simulink model "nms_3Dmodel_forward"  (R2017b)
settings: Solver=VariableStepAuto  StartTime=0.0  StopTime=t_end  FixedStep=1e-4  MinStep=1e-9  RelTol=1e-2  AbsTol=1e-3  EnableMultiTasking=on
InitFcn:
  | runScripts;
values from neighbouring files (symbols this model uses):
  ankle_height = 0.08    [nms_MechInit.m]
  ankleIMP = param(91+length(paramIC_opt):93+length(paramIC_opt))    [runScripts.m]
  c = 0.05    [IID_nms_MechInit.m]    (also in nms_MechInit.m)
  c_jointstop = 0.3 / (pi/180)    (= 17.1887338539)    [IID_nms_MechInit.m]    (also in nms_MechInit.m)
  CPG_On = 0    [setCPGPar.m]    (also in setCPGPar_inv.m = 1)
  CtrlPar_FP = [alpha0 alpha_cd alpha_cv]    [setCtrlPar.m]
  CtrlPar_FP_R = [R_hipR0 R_hipR_cd R_hipR_cv]    [setCtrlPar.m]
  CtrlPar_LL = l_clr    [setCtrlPar.m]
  CtrlPar_Side = [beta_cd  beta_cv]    [setCtrlPar.m]
  CtrlPar_St = [StPreStim St_M1 St_M2 St_M3 St_M4 St_M5 St_M11]    [setCtrlPar.m]
  CtrlPar_St_R = [R_StPreStim R_St_M1 R_St_M3 R_St_M4]    [setCtrlPar.m]
  CtrlPar_Sw = [SwPreStim SwPhasePari SwPhaseParii SwCtrlPar_H SwCtrlPar_A      SwCtrlPar_Ki SwCtrlPar_Kii SwCtrlPar_Kiii SwCtrlPar_StP]    [setCtrlPar.m]
  CtrlPar_Sw_R = [R_SwPreStim R_Sw_M6]    [setCtrlPar.m]
  CtrlPar_theta0 = parBlCtrl(1)      *1*pi/180    [setCtrlPar.m]
  CtrlPar_Tr = [Tr_St_sup Tr_Sw]    [setCtrlPar.m]
  CtrlPar_Tr_R = [R_Tr_St_sup R_Tr_Sw]    [setCtrlPar.m]
  D12_F = 0.16    [IID_nms_MechInit.m]    (also in nms_MechInit.m)
  D12_S = L_S    (= 0.5)    [IID_nms_MechInit.m]    (also in nms_MechInit.m = 0.46)
  D12_T = L_T    (= 0.5)    [IID_nms_MechInit.m]    (also in nms_MechInit.m = 0.46)
  D12z_T = 0.1* scalorFactor    (= 0.1)    [nms_MechInit.m]
  D13_F = 0.20    (= 0.2)    [IID_nms_MechInit.m]    (also in nms_MechInit.m)
  D1G_F = 0.14    [IID_nms_MechInit.m]    (also in nms_MechInit.m)
  D1G_HAT = 0.35    [IID_nms_MechInit.m]    (also in nms_MechInit.m)
  D1G_S = 0.3    [IID_nms_MechInit.m]    (also in nms_MechInit.m = 0.28)
  D1G_T = 0.3    [IID_nms_MechInit.m]    (also in nms_MechInit.m = 0.28)
  D1Gy_F = ankle_height*D1G_F/D12_F    (= 0.07)    [nms_MechInit.m]
  d_fBall = 0.1    [nms_MechInit.m]
  d_fHeel = 0.05    [nms_MechInit.m]
  DeltaThRef = 5e-3    (= 0.005)    [IID_nms_MechInit.m]    (also in nms_MechInit.m)
  Dist_LM23_PH = 0    [setDistPar.m]
  Dist_LM34_PH = 0    [setDistPar.m]
  Dist_On = 1    [IID_setDistPar.m]    (also in setDistPar.m)
  Dist_PDur = 0.15    [IID_setDistPar.m]    (also in setDistPar.m)
  Dist_RM23_PH = 0    [setDistPar.m]
  Dist_RM34_PH = 0    [setDistPar.m]
  Dist_StartTime = 15    [IID_setDistPar.m]    (also in setDistPar.m)
  Dist_xyzHAT_front_PH = 0    [setDistPar.m]
  Dist_xyzHAT_sag_PH = 0    [IID_setDistPar.m]    (also in setDistPar.m)
  Dist_xyzLAnkle_PH = 0    [setDistPar.m]
  Dist_xyzRAnkle_PH = 0    [setDistPar.m]
  eref = 0.04    [IID_nms_MechInit.m]    (also in nms_MechInit.m)
  FmaxBFSH = 350    [nms_MechInit.m]
  FmaxGAS = 1500    [IID_nms_MechInit.m]    (also in nms_MechInit.m)
  FmaxGLU = 1500    [IID_nms_MechInit.m]    (also in nms_MechInit.m)
  FmaxHAB = 3000    [nms_MechInit.m]
  FmaxHAD = 4500    [nms_MechInit.m]
  FmaxHAM = 3000    [IID_nms_MechInit.m]    (also in nms_MechInit.m)
  FmaxHFL = 2000    [IID_nms_MechInit.m]    (also in nms_MechInit.m)
  FmaxRF = 1200    [nms_MechInit.m]
  FmaxSOL = 4000    [IID_nms_MechInit.m]    (also in nms_MechInit.m)
  FmaxTA = 800    [IID_nms_MechInit.m]    (also in nms_MechInit.m)
  FmaxVAS = 6000    [IID_nms_MechInit.m]    (also in nms_MechInit.m)
  In_F = 0.005    [IID_nms_MechInit.m]    (also in nms_MechInit.m)
  In_HAT = 3    [IID_nms_MechInit.m]    (also in nms_MechInit.m = 2.5)
  In_S = 0.05    [IID_nms_MechInit.m]    (also in nms_MechInit.m)
  In_T = 0.15    [IID_nms_MechInit.m]    (also in nms_MechInit.m)
  init_a_tgt = 70*pi/180    (= 1.2217304764)    [setInitPar.m]
  init_a_tgtR = 90*pi/180    (= 1.57079632679)    [setInitPar.m]
  Inx_F = 0.0007    [nms_MechInit.m]
  Inx_HAT = 1.0    (= 1)    [nms_MechInit.m]
  Inx_S = 0.003    [nms_MechInit.m]
  Inx_T = 0.03    [nms_MechInit.m]
  Iny_F = 0.005    [nms_MechInit.m]
  Iny_HAT = 4.0    (= 4)    [nms_MechInit.m]
  Iny_S = 0.05    [nms_MechInit.m]
  Iny_T = 0.15    [nms_MechInit.m]
  K = 5    [IID_nms_MechInit.m]    (also in nms_MechInit.m)
  k_gn = k_gn/2    (= 39240)    [nms_MechInit.m]
  k_gt = k_gt/2    (= 3924)    [nms_MechInit.m]
  k_pressure = m_HAT * 9.81 / DeltaThRef    (= 104967)    [IID_nms_MechInit.m]    (also in nms_MechInit.m)
  leg_l = [D12_T D12_S]    [nms_MechInit.m]
  LongDelay = 0.020    (= 0.02)    [IID_setCtrlPar.m]    (also in nms_MechInit.m = 0.01)
  LongLoopDelay = 0.030    (= 0.03)    [nms_MechInit.m]
  loptBFSH = 0.12    [nms_MechInit.m]
  loptGAS = 0.05    [IID_nms_MechInit.m]    (also in nms_MechInit.m)
  loptGLU = 0.11    [IID_nms_MechInit.m]    (also in nms_MechInit.m)
  loptHAB = 0.09    [nms_MechInit.m]
  loptHAD = 0.10    (= 0.1)    [nms_MechInit.m]
  loptHAM = 0.10    (= 0.1)    [IID_nms_MechInit.m]    (also in nms_MechInit.m)
  loptHFL = 0.11    [IID_nms_MechInit.m]    (also in nms_MechInit.m)
  loptRF = 0.08    [nms_MechInit.m]
  loptSOL = 0.04    [IID_nms_MechInit.m]    (also in nms_MechInit.m)
  loptTA = 0.06    [IID_nms_MechInit.m]    (also in nms_MechInit.m)
  loptVAS = 0.08    [IID_nms_MechInit.m]    (also in nms_MechInit.m)
  lslackBFSH = 0.10    (= 0.1)    [nms_MechInit.m]
  lslackGAS = 0.40    (= 0.4)    [IID_nms_MechInit.m]    (also in nms_MechInit.m)
  lslackGLU = 0.13    [IID_nms_MechInit.m]    (also in nms_MechInit.m)
  lslackHAB = 0.07    [nms_MechInit.m]
  lslackHAD = 0.18    [nms_MechInit.m]
  lslackHAM = 0.31    [IID_nms_MechInit.m]    (also in nms_MechInit.m)
  lslackHFL = 0.10    (= 0.1)    [IID_nms_MechInit.m]    (also in nms_MechInit.m)
  lslackRF = 0.35    [nms_MechInit.m]
  lslackSOL = 0.26    [IID_nms_MechInit.m]    (also in nms_MechInit.m)
  lslackTA = 0.24    [IID_nms_MechInit.m]    (also in nms_MechInit.m)
  lslackVAS = 0.23    [IID_nms_MechInit.m]    (also in nms_MechInit.m)
  m_F = 1.25    [IID_nms_MechInit.m]    (also in nms_MechInit.m)
  m_HAT = 53.5    [IID_nms_MechInit.m]    (also in nms_MechInit.m)
  m_S = 3.5    [IID_nms_MechInit.m]    (also in nms_MechInit.m)
  m_T = 8.5    [IID_nms_MechInit.m]    (also in nms_MechInit.m)
  m_Total = m_F*2+m_S*2+m_T*2+m_HAT    (= 80)    [IID_nms_MechInit.m]    (also in nms_MechInit.m)
  massBFSH = 2    [nms_MechInit.m]
  massGAS = 0.45    [IID_nms_MechInit.m]    (also in nms_MechInit.m)
  massGLU = 1.4    [IID_nms_MechInit.m]    (also in nms_MechInit.m)
  massHAB = 1.145    [nms_MechInit.m]
  massHAD = 1.91    [nms_MechInit.m]
  massHAM = 1.82    [IID_nms_MechInit.m]    (also in nms_MechInit.m)
  massHFL = 1.87    [IID_nms_MechInit.m]    (also in nms_MechInit.m)
  massRF = 1    [nms_MechInit.m]
  massSOL = 1.36    [IID_nms_MechInit.m]    (also in nms_MechInit.m)
  massTA = 0.29    [IID_nms_MechInit.m]    (also in nms_MechInit.m)
  massVAS = 2.91    [IID_nms_MechInit.m]    (also in nms_MechInit.m)
  MidDelay = 0.010    (= 0.01)    [IID_setCtrlPar.m]    (also in nms_MechInit.m = 0.005)
  mu_slide = 0.8    [IID_nms_MechInit.m]    (also in nms_MechInit.m)
  mu_stick = 0.9    [IID_nms_MechInit.m]    (also in nms_MechInit.m)
  N = 1.5    [IID_nms_MechInit.m]    (also in cmaes_parfor.m = size(x,1); nms_MechInit.m)
  phi12_LowLimit = 70*pi/180    (= 1.2217304764)    [IID_nms_MechInit.m]    (also in nms_MechInit.m)
  phi12_UpLimit = 130*pi/180    (= 2.26892802759)    [IID_nms_MechInit.m]    (also in nms_MechInit.m)
  phi23_UpLimit = 175*pi/180    (= 3.05432619099)    [IID_nms_MechInit.m]    (also in nms_MechInit.m)
  phi34_UpLimit = 230*pi/180    (= 4.01425727959)    [IID_nms_MechInit.m]    (also in nms_MechInit.m)
  phi34R_LowLimit = -15*pi/180    (= -0.261799387799)    [nms_MechInit.m]
  ... (+115 more)
undefined symbols (not defined in the file or in its folder): Control_type, Fs_prosthesis, magnitude, sgn
libraries: mblibv1 x104, simulink x54, simulink_extras x38, nmc x30, NMCCPG_Library x17, powerlib_meascontrol x5
(part 3 of 17)

== system nms_3Dmodel_forward/CPG ==
  note: CPG State Observer
      | Learning Center
      | Learns the signals of all sensors
      | If signals are prelearned, only loads the signals
      |
      | CPG Output
      | Estimates rate of change (roc at all instances of various time model
      | Becomes active after signals are saved or loaded
      |
      | Saver
      | Saves signals to workspace after learning is done
      |
      | Etc
      | Creates signals necessary in CPG model
  CPG Output : Subsystem
  Etc : Subsystem
  Learning center : Subsystem
  Saver : Subsystem  Commented=on

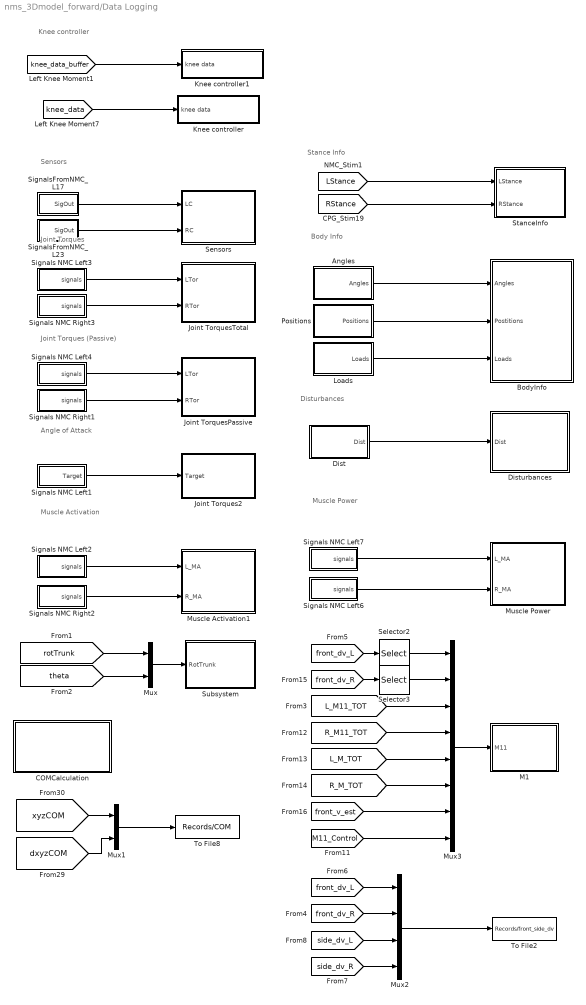
== system nms_3Dmodel_forward/Data Logging ==
  note: Sensors
  note: Stance Info
  note: Muscle Activation
  note: Joint Torques
  note: Disturbances
  note: Angle of Attack
  note: Body Info
  note: Joint Torques (Passive)
  note: Muscle Power
  note: Knee controller
  Angles : Subsystem
  BodyInfo : Subsystem
  "COMCalculation " : Subsystem
  Dist : Subsystem
  Disturbances : Subsystem
  Joint Torques2 : Subsystem
  Joint TorquesPassive : Subsystem
  Joint TorquesTotal : Subsystem
  Knee controller : Subsystem
  Knee controller1 : Subsystem
  Loads : Subsystem
  M1 : Subsystem
  Muscle Activation1 : Subsystem
  Muscle Power : Subsystem
  Mux : Mux  Inputs=2
  Mux1 : Mux  Inputs=2
  Mux2 : Mux
  Mux3 : Mux  Inputs=8
  Positions : Subsystem
  Selector2 : Selector  InputPortWidth=2  IndexOptions=Index vector (dialog)  Indices=[2]  OutputSizes=1
  Selector3 : Selector  InputPortWidth=2  IndexOptions=Index vector (dialog)  Indices=[2]  OutputSizes=1
  Sensors : Subsystem
  Signals NMC Left1 : Subsystem
  Signals NMC Left2 : Subsystem
  Signals NMC Left3 : Subsystem
  Signals NMC Left4 : Subsystem
  Signals NMC Left6 : Subsystem
  Signals NMC Left7 : Subsystem
  Signals NMC Right1 : Subsystem
  Signals NMC Right2 : Subsystem
  Signals NMC Right3 : Subsystem
  SignalsFromNMC_L17 : Subsystem  mask{LorR='L', Add=''}
      mask prompts: LorR "Right or Left"; Add "Addition"
      mask init:
      | blk = gcb;
      | set_param([gcb '/From'],'GotoTag',[LorR,'FmGLU',Add]);
      | set_param([gcb '/From1'],'GotoTag',[LorR,'FmHAM',Add]);
      | set_param([gcb '/From2'],'GotoTag',[LorR,'FmVAS',Add]);
      | set_param([gcb '/From3'],'GotoTag',[LorR,'LceBFSH',Add]);
      | set_param([gcb '/From4'],'GotoTag',[LorR,'FmGAS',Add]);
      | 
      | set_param([gcb '/From5'],'GotoTag',[LorR,'FmSOL',Add]);
      | set_param([gcb '/From6'],'GotoTag',[LorR,'LceTA',Add]);
      | set_param([gcb '/From7'],'GotoTag',[LorR,'LceRF',Add]);
      | set_param([gcb '/From8'],'GotoTag',[LorR,'VceRF',Add]);
      | set_param([gcb '/From9'],'GotoTag',[LorR,'LceHAM',Add]);
      | 
      | set_param([gcb '/From10'],'GotoTag',[LorR,'VceHAM',Add]);
      | set_param([gcb '/From11'],'GotoTag',[LorR,'VceVAS',Add]);
      | set_param([gcb '/From12'],'GotoTag',[LorR,'VceBFSH',Add]);
      | set_param([gcb '/From13'],'GotoTag',[LorR,'LceHFL',Add]);
      | set_param([gcb '/From14'],'GotoTag',[LorR,'LceGLU',Add]);
      | 
      | set_param([gcb '/From15'],'GotoTag',[LorR,'LceVAS',Add]);
      | set_param([gcb '/From16'],'GotoTag',[LorR,'FmHAB',Add]);
      | set_param([gcb '/From17'],'GotoTag',[LorR,'LceHAD',Add]);
      | set_param([gcb '/From18'],'GotoTag',[LorR,'LceHAB',Add]);
  SignalsFromNMC_L23 : Subsystem  mask{LorR='R', Add=''}
      mask prompts: LorR "Right or Left"; Add "Addition"
      mask init: same as nms_3Dmodel_forward/Data Logging/SignalsFromNMC_L17
  StanceInfo : Subsystem
  Subsystem : Subsystem
  To File2 : ToFile  Filename=Records/front_side_dv
  To File8 : ToFile  Filename=Records/COM
  wires:
  SignalsFromNMC_L17/1(SigOut) -> Sensors/1(LC)
  SignalsFromNMC_L23/1(SigOut) -> Sensors/2(RC)
  Signals NMC Right2/1(signals) -> Muscle Activation1/2(R_MA)
  Signals NMC Left2/1(signals) -> Muscle Activation1/1(L_MA)
  Signals NMC Left3/1(signals) -> Joint TorquesTotal/1(LTor)
  Signals NMC Right3/1(signals) -> Joint TorquesTotal/2(RTor)
  Angles/1(Angles) -> BodyInfo/1(Angles)
  Positions/1(Positions) -> BodyInfo/2(Postitions)
  [LStance] -> StanceInfo/1(LStance)
  [RStance] -> StanceInfo/2(RStance)
  Loads/1(Loads) -> BodyInfo/3(Loads)
  Signals NMC Left1/1(Target) -> Joint Torques2/1(Target)
  Dist/1(Dist) -> Disturbances/1(Dist)
  [rotTrunk] -> Mux/1
  [theta] -> Mux/2
  Signals NMC Left4/1(signals) -> Joint TorquesPassive/1(LTor)
  Signals NMC Right1/1(signals) -> Joint TorquesPassive/2(RTor)
  Signals NMC Left6/1(signals) -> Muscle Power/2(R_MA)
  Signals NMC Left7/1(signals) -> Muscle Power/1(L_MA)
  Mux/1 -> Subsystem/1(RotTrunk)
  [dxyzCOM] -> Mux1/2
  [xyzCOM] -> Mux1/1
  Mux1/1 -> To File8/1
  Selector2/1 -> Mux3/1
  [front_dv_L] -> Selector2/1
  [L_M_TOT] -> Mux3/5
  [R_M_TOT] -> Mux3/6
  [L_M11_TOT] -> Mux3/3
  [R_M11_TOT] -> Mux3/4
  [front_dv_R] -> Selector3/1
  Selector3/1 -> Mux3/2
  Mux3/1 -> M1/1(M11)
  [M11_Control] -> Mux3/8
  [front_v_est] -> Mux3/7
  [side_dv_R] -> Mux2/4
  [front_dv_R] -> Mux2/2
  [side_dv_L] -> Mux2/3
  [front_dv_L] -> Mux2/1
  Mux2/1 -> To File2/1
  [knee_data] -> Knee controller/1(knee data)
  [knee_data_buffer] -> Knee controller1/1(knee data)

== system nms_3Dmodel_forward/Disturbances ==
  Clock : Clock
  Compare To Constant : simulink/Logic and Bit Operations/Compare To Constant  relop=>  const=Dist_StartTime  OutDataTypeStr=boolean
  Compare To Constant1 : simulink/Logic and Bit Operations/Compare To Constant  relop===  const=0  OutDataTypeStr=boolean
  Compare To Constant2 : simulink/Logic and Bit Operations/Compare To Constant  relop===  const=1  OutDataTypeStr=boolean
  Compare To Constant3 : simulink/Logic and Bit Operations/Compare To Constant  relop=<  const=Dist_PDur  OutDataTypeStr=boolean
  Constant : Constant  Value=zeros(8,1)
  Constant1 : Constant  Value=Dist_On
  Constant2 : Constant  Value=[Dist_xyzHAT_sag_PH;Dist_xyzHAT_front_PH;Dist_xyzLAnkle_PH;Dist_xyzRAnkle_PH;Dist_LM34_PH;Dist_RM34_PH;Dist_LM23_PH;Dist_RM23_PH]
  Disturbances : Subsystem
  Integrator : Integrator
  Logical Operator : Logic  Inputs=4  AllPortsSameDT=off  OutDataTypeStr=boolean
  Logical Operator1 : Logic  AllPortsSameDT=off  OutDataTypeStr=boolean
  SampleAndHold : Subsystem
  Start Disturbance torques onces CPG is turned on : Switch  Criteria=u2 ~= 0
  Transport Delay1 : TransportDelay  DelayTime=0.01
  wires:
  Constant1/1 -> Logical Operator/2
  Compare To Constant/1 -> Logical Operator/1
  Constant2/1 -> Start Disturbance torques onces CPG is turned on/1
  Start Disturbance torques onces CPG is turned on/1 -> Disturbances/1(Dist)
  Constant/1 -> Start Disturbance torques onces CPG is turned on/3
  Clock/1 -> Compare To Constant/1
  Compare To Constant1/1 -> Logical Operator/3
  [LStance] -> Compare To Constant1/1, Transport Delay1/1
  Compare To Constant2/1 -> Logical Operator/4
  Logical Operator1/1 -> Start Disturbance torques onces CPG is turned on/2
  Transport Delay1/1 -> Compare To Constant2/1
  Integrator/1 -> Compare To Constant3/1
  Compare To Constant3/1 -> Logical Operator1/2
  SampleAndHold/1(Out) -> Logical Operator1/1, Integrator/1
  Logical Operator/1 -> SampleAndHold/1(Sample), SampleAndHold/2(Value)

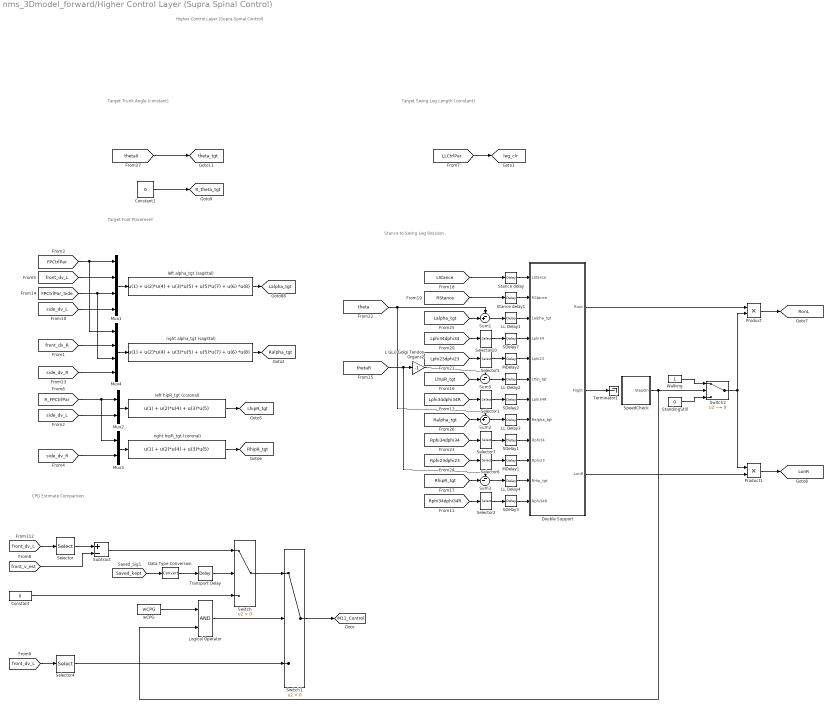
== system nms_3Dmodel_forward/Higher Control Layer (Supra Spinal Control) ==
  note: Target Foot Placement
  note: Target Swing Leg Length
      | (constant)
  note: Stance to Swing Leg Decision
  note: Target Trunk Angle
      | (constant)
  note: Higher Control Layer
      | (Supra Spinal Control)
  note: CPG Estimate Comparison
  Constant : Constant  Value=0
  Constant1 : Constant  Value=0
  Data Type Conversion : DataTypeConversion
  Double Support : Subsystem
  L GLU Golgi Tendon Organs2 : Gain  Gain=-1
  LL Delay1 : TransportDelay  DelayTime=LongLoopDelay/2  InitialOutput=init_a_tgt
  LL Delay2 : TransportDelay  DelayTime=LongLoopDelay/2
  LL Delay3 : TransportDelay  DelayTime=LongLoopDelay/2  InitialOutput=init_a_tgt
  LL Delay4 : TransportDelay  DelayTime=LongLoopDelay/2
  Logical Operator : Logic  AllPortsSameDT=off  OutDataTypeStr=boolean
  MDelay1 : TransportDelay  DelayTime=MidDelay
  MDelay2 : TransportDelay  DelayTime=MidDelay
  Mux1 : Mux
  Mux2 : Mux  Inputs=2
  Mux3 : Mux  Inputs=2
  Mux4 : Mux
  Product : Product
  Product1 : Product
  SDelay{1..3,7} (4 alike) : TransportDelay  DelayTime=ShortDelay
  Selector : Selector  InputPortWidth=2  IndexOptions=Index vector (dialog)  Indices=[2]  OutputSizes=1
  Selector{1..2,5..7,10} (6 alike) : Selector  InputPortWidth=2  IndexOptions=Index vector (dialog)  Indices=1  OutputSizes=1
  Selector4 : Selector  InputPortWidth=2  IndexOptions=Index vector (dialog)  Indices=[2]  OutputSizes=1
  SpeedCheck : Subsystem
  Stance delay : TransportDelay  DelayTime=MidDelay
  Stance delay1 : TransportDelay  DelayTime=MidDelay
  StandingStill : Constant  Value=0
  Subtract : Sum  Inputs=+-
  Sum1 : Sum  Inputs=-+|
  Sum2 : Sum  Inputs=-+|
  Sum3 : Sum  Inputs=--|
  Sum5 : Sum  Inputs=--|
  Switch : Switch  Criteria=u2 > Threshold
  Switch1 : Switch  Criteria=u2 > Threshold
  Switch2 : Switch  Criteria=u2 ~= 0
  Terminator1 : Terminator
  Transport Delay : TransportDelay  DelayTime=0.1
  Walking : Constant
  left alpha_tgt (sagittal) : Fcn  Expr=u(1) + u(2)*u(4) + u(3)*u(5) + u(5)*u(7) + u(6) *u(8)
  left hipR_tgt (coronal) : Fcn  Expr=u(1) + u(2)*u(4) + u(3)*u(5)
  right alpha_tgt (sagittal) : Fcn  Expr=u(1) + u(2)*u(4) + u(3)*u(5) + u(5)*u(7) + u(6) *u(8)
  right hipR_tgt (coronal) : Fcn  Expr=u(1) + u(2)*u(4) + u(3)*u(5)
  wCPG : Constant  Value=wCPG
  tag scope: Lalpha_tgt=global, LhipR_tgt=global, LonR=global, M11_Control=global, R_theta_tgt=global, Ralpha_tgt=global, RhipR_tgt=global, RonL=global, leg_clr=global, theta_tgt=global
  wires:
  left alpha_tgt (sagittal)/1 -> [Lalpha_tgt]
  right alpha_tgt (sagittal)/1 -> [Ralpha_tgt]
  left hipR_tgt (coronal)/1 -> [LhipR_tgt]
  right hipR_tgt (coronal)/1 -> [RhipR_tgt]
  [LLCtrlPar] -> [leg_clr]
  [Lphi34dphi34] -> Selector10/1
  [Lphi23dphi23] -> Selector5/1
  Selector10/1 -> SDelay7/1
  Selector5/1 -> MDelay2/1
  [Rphi34dphi34] -> Selector7/1
  [Rphi23dphi23] -> Selector6/1
  Selector7/1 -> SDelay1/1
  Selector6/1 -> MDelay1/1
  Double Support/3(LonR) -> Product1/2
  Stance delay/1 -> Double Support/1(LStance)
  Stance delay1/1 -> Double Support/2(RStance)
  Double Support/1(RonL) -> Product/1
  [LStance] -> Stance delay/1
  [RStance] -> Stance delay1/1
  Double Support/2(Flight) -> Terminator1/1
  LL Delay1/1 -> Double Support/3(Lalpha_tgt)
  LL Delay3/1 -> Double Support/8(Ralpha_tgt)
  SDelay7/1 -> Double Support/4(Lphi34)
  SDelay1/1 -> Double Support/9(Rphi34)
  MDelay2/1 -> Double Support/5(Lphi23)
  MDelay1/1 -> Double Support/10(Rphi23)
  Sum1/1 -> LL Delay1/1
  [Lalpha_tgt] -> Sum1/2
  [theta] -> Sum1/1, Sum2/1
  [Ralpha_tgt] -> Sum2/2
  Sum2/1 -> LL Delay3/1
  [Lphi34dphi34R] -> Selector1/1
  Selector1/1 -> SDelay2/1
  SDelay2/1 -> Double Support/7(Lphi34R)
  LL Delay2/1 -> Double Support/6(LHip_tgt)
  Sum5/1 -> LL Delay2/1
  [LhipR_tgt] -> Sum5/2
  [thetaR] -> L GLU Golgi Tendon Organs2/1, Sum3/1
  L GLU Golgi Tendon Organs2/1 -> Sum5/1
  [Rphi34dphi34R] -> Selector2/1
  Selector2/1 -> SDelay3/1
  SDelay3/1 -> Double Support/12(Rphi34R)
  LL Delay4/1 -> Double Support/11(RHip_tgt)
  Sum3/1 -> LL Delay4/1
  [RhipR_tgt] -> Sum3/2
  [theta0] -> [theta_tgt]
  Constant1/1 -> [R_theta_tgt]
  Mux1/1 -> left alpha_tgt (sagittal)/1
  [FPCtrlPar] -> Mux4/1, Mux1/1
  [front_dv_L] -> Mux1/2
  Mux4/1 -> right alpha_tgt (sagittal)/1
  [front_dv_R] -> Mux4/2
  Mux2/1 -> left hipR_tgt (coronal)/1
  Mux3/1 -> right hipR_tgt (coronal)/1
  [R_FPCtrlPar] -> Mux3/1, Mux2/1
  [side_dv_L] -> Mux2/2
  [side_dv_R] -> Mux3/2
  [front_dv_L] -> Selector/1
  Selector/1 -> Subtract/1
  [front_v_est] -> Subtract/2
  Subtract/1 -> Switch/1
  [Saved_kept] -> Data Type Conversion/1
  Switch/1 -> Switch1/1
  Transport Delay/1 -> Switch/2
  Constant/1 -> Switch/3
  Data Type Conversion/1 -> Transport Delay/1
  [front_dv_L] -> Selector4/1
  Selector4/1 -> Switch1/3
  Switch1/1 -> [M11_Control]
  wCPG/1 -> Logical Operator/1
  Product/1 -> [RonL]
  Product1/1 -> [LonR]
  Walking/1 -> Switch2/1
  StandingStill/1 -> Switch2/3
  Switch2/1 -> Product/2, Product1/1
  Logical Operator/1 -> Switch1/2
  SpeedCheck/1(StepOn) -> Logical Operator/2, Switch2/2
  [side_dv_L] -> Mux1/4
  [side_dv_R] -> Mux4/4
  [FPCtrlPar_Side] -> Mux4/3, Mux1/3

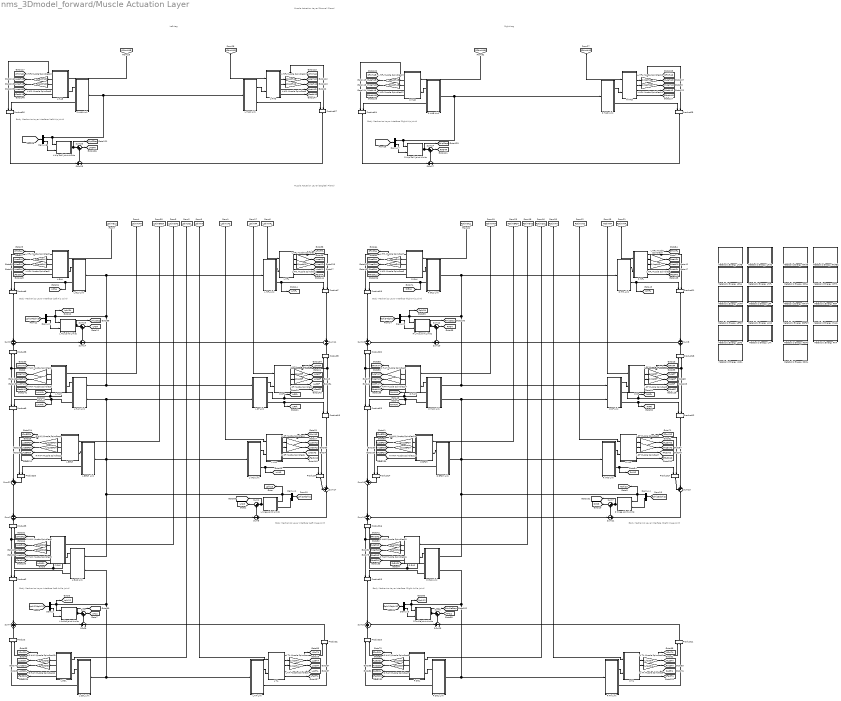
== system nms_3Dmodel_forward/Muscle Actuation Layer ==
  note: Muscle Actuation Layer
      | (Sagittal Plane)
  note: Body Mechanics Layer
      | Interface (Left Hip Joint)
  note: Body Mechanics Layer
      | Interface (Left Knee Joint)
  note: Body Mechanics Layer
      | Interface (Left Ankle Joint)
  note: Body Mechanics Layer
      | Interface (Right Hip Joint)
  note: Body Mechanics Layer
      | Interface (Right Knee Joint)
  note: Body Mechanics Layer
      | Interface (Right Ankle Joint)
  note: Left Leg
  note: Body Mechanics Layer
      | Interface (Left Hip Joint)
  note: Body Mechanics Layer
      | Interface (Right Hip Joint)
  note: Right Leg
  note: Muscle Actuation Layer
      | (Coronal Plane)
  Demux{,1..7} (8 alike) : Demux  Outputs=2
  F GAS : Subsystem
  L Ankle Joint Limits : Subsystem
  L BFSH : Subsystem
  L BFSH Link : Subsystem
  L GAS Link : Subsystem
  L GLU : Subsystem
  L GLU Link : Subsystem
  L HAB : Subsystem
  L HAB Link : Subsystem
  L HAD : Subsystem
  L HAD Link : Subsystem
  L HAM : Subsystem
  L HAM Link : Subsystem
  L HFL : Subsystem
  L HFL Muscle Spindles{,1,4..5} (4 alike) : Gain  Gain=1/loptHFL
  L HFL Muscle Spindles{9..10,12..13} (4 alike) : Gain  Gain=1/loptHAB
  L HFL Muscle Spindles{8,11,14..15} (4 alike) : Gain  Gain=1/loptHAD
  L HFL Muscle Spindles{2..3,6..7} (4 alike) : Gain  Gain=1/loptGLU
  L HFL Link : Subsystem
  L Hip Joint Limits : Subsystem
  L Hip Roll Joint Limits : Subsystem
  L Knee Joint Limits : Subsystem
  L RF Muscle Spindles{,1..3} (4 alike) : Gain  Gain=1/loptRF
  L RF Muscle Spindles{4..7} (4 alike) : Gain  Gain=1/loptVAS
  L RF Link : Subsystem
  L SOL : Subsystem
  L SOL Link : Subsystem
  L TA : Subsystem
  L TA Muscle Spindles{,1..3} (4 alike) : Gain  Gain=1/loptTA
  L TA Link : Subsystem
  L VAS : Subsystem
  L VAS Link : Subsystem
  Metabolic Energy LBFSH : Subsystem  mask{side='L', muscle='BFSH'}
      mask prompts: side "What Side (R/L)?"; muscle "What Muscle?"
      mask init:
      | blk = gcb;
      | 
      | set_param([gcb '/From1'],'GotoTag',[side,'Act',muscle]);
      | set_param([gcb '/From2'],'GotoTag',[side,'Stim',muscle]);
      | set_param([gcb '/From3'],'GotoTag',[side,'Lce',muscle]);
      | set_param([gcb '/From4'],'GotoTag',[side,'Vce',muscle]);
      | set_param([gcb '/From5'],'GotoTag',[side,'Fm',muscle]);
      | set_param([gcb '/From6'],'GotoTag',[side,'Fact',muscle]);
      | 
      | set_param([gcb '/Goto1'],'GotoTag',[side,'Energy',muscle]);
      | 
      | set_param([gcb '/Constant'],'Value',['lopt',muscle]);
      | set_param([gcb '/Constant1'],'Value',['mass',muscle]);
      | set_param([gcb '/Constant2'],'Value',['t1f',muscle]);
  Metabolic Energy LGAS : Subsystem  mask{side='L', muscle='GAS'}
      mask prompts: side "What Side (R/L)?"; muscle "What Muscle?"
      mask init: same as nms_3Dmodel_forward/Muscle Actuation Layer/Metabolic Energy LBFSH
  Metabolic Energy LGLU : Subsystem  mask{side='L', muscle='GLU'}
      mask prompts: side "What Side (R/L)?"; muscle "What Muscle?"
      mask init: same as nms_3Dmodel_forward/Muscle Actuation Layer/Metabolic Energy LBFSH
  Metabolic Energy LHAB : Subsystem  mask{side='L', muscle='HAB'}
      mask prompts: side "What Side (R/L)?"; muscle "What Muscle?"
      mask init: same as nms_3Dmodel_forward/Muscle Actuation Layer/Metabolic Energy LBFSH
  Metabolic Energy LHAD : Subsystem  mask{side='L', muscle='HAD'}
      mask prompts: side "What Side (R/L)?"; muscle "What Muscle?"
      mask init: same as nms_3Dmodel_forward/Muscle Actuation Layer/Metabolic Energy LBFSH
  Metabolic Energy LHAM : Subsystem  mask{side='L', muscle='HAM'}
      mask prompts: side "What Side (R/L)?"; muscle "What Muscle?"
      mask init: same as nms_3Dmodel_forward/Muscle Actuation Layer/Metabolic Energy LBFSH
  Metabolic Energy LHFL : Subsystem  mask{side='L', muscle='HFL'}
      mask prompts: side "What Side (R/L)?"; muscle "What Muscle?"
      mask init: same as nms_3Dmodel_forward/Muscle Actuation Layer/Metabolic Energy LBFSH
  Metabolic Energy LRF : Subsystem  mask{side='L', muscle='RF'}
      mask prompts: side "What Side (R/L)?"; muscle "What Muscle?"
      mask init: same as nms_3Dmodel_forward/Muscle Actuation Layer/Metabolic Energy LBFSH
  Metabolic Energy LSOL : Subsystem  mask{side='L', muscle='SOL'}
      mask prompts: side "What Side (R/L)?"; muscle "What Muscle?"
      mask init: same as nms_3Dmodel_forward/Muscle Actuation Layer/Metabolic Energy LBFSH
  Metabolic Energy LTA : Subsystem  mask{side='L', muscle='TA'}
      mask prompts: side "What Side (R/L)?"; muscle "What Muscle?"
      mask init: same as nms_3Dmodel_forward/Muscle Actuation Layer/Metabolic Energy LBFSH
  Metabolic Energy LVAS : Subsystem  mask{side='L', muscle='VAS'}
      mask prompts: side "What Side (R/L)?"; muscle "What Muscle?"
      mask init: same as nms_3Dmodel_forward/Muscle Actuation Layer/Metabolic Energy LBFSH
  Metabolic Energy RBFSH : Subsystem  mask{side='R', muscle='BFSH'}
      mask prompts: side "What Side (R/L)?"; muscle "What Muscle?"
      mask init: same as nms_3Dmodel_forward/Muscle Actuation Layer/Metabolic Energy LBFSH
  Metabolic Energy RGAS : Subsystem  mask{side='R', muscle='GAS'}
      mask prompts: side "What Side (R/L)?"; muscle "What Muscle?"
      mask init: same as nms_3Dmodel_forward/Muscle Actuation Layer/Metabolic Energy LBFSH
  Metabolic Energy RGLU : Subsystem  mask{side='R', muscle='GLU'}
      mask prompts: side "What Side (R/L)?"; muscle "What Muscle?"
      mask init: same as nms_3Dmodel_forward/Muscle Actuation Layer/Metabolic Energy LBFSH
  Metabolic Energy RHAB : Subsystem  mask{side='R', muscle='HAB'}
      mask prompts: side "What Side (R/L)?"; muscle "What Muscle?"
      mask init: same as nms_3Dmodel_forward/Muscle Actuation Layer/Metabolic Energy LBFSH
  Metabolic Energy RHAB1 : Subsystem  mask{side='R', muscle='HAD'}
      mask prompts: side "What Side (R/L)?"; muscle "What Muscle?"
      mask init: same as nms_3Dmodel_forward/Muscle Actuation Layer/Metabolic Energy LBFSH
  Metabolic Energy RHAM : Subsystem  mask{side='R', muscle='HAM'}
      mask prompts: side "What Side (R/L)?"; muscle "What Muscle?"
      mask init: same as nms_3Dmodel_forward/Muscle Actuation Layer/Metabolic Energy LBFSH
  Metabolic Energy RHFL : Subsystem  mask{side='R', muscle='HFL'}
      mask prompts: side "What Side (R/L)?"; muscle "What Muscle?"
      mask init: same as nms_3Dmodel_forward/Muscle Actuation Layer/Metabolic Energy LBFSH
  Metabolic Energy RRF : Subsystem  mask{side='R', muscle='RF'}
      mask prompts: side "What Side (R/L)?"; muscle "What Muscle?"
      mask init: same as nms_3Dmodel_forward/Muscle Actuation Layer/Metabolic Energy LBFSH
  Metabolic Energy RSOL : Subsystem  mask{side='R', muscle='SOL'}
      mask prompts: side "What Side (R/L)?"; muscle "What Muscle?"
      mask init: same as nms_3Dmodel_forward/Muscle Actuation Layer/Metabolic Energy LBFSH
  Metabolic Energy RTA : Subsystem  mask{side='R', muscle='TA'}
      mask prompts: side "What Side (R/L)?"; muscle "What Muscle?"
      mask init: same as nms_3Dmodel_forward/Muscle Actuation Layer/Metabolic Energy LBFSH
  Metabolic Energy RVAS : Subsystem  mask{side='R', muscle='VAS'}
      mask prompts: side "What Side (R/L)?"; muscle "What Muscle?"
      mask init: same as nms_3Dmodel_forward/Muscle Actuation Layer/Metabolic Energy LBFSH
  Product{,1..27} (28 alike) : Product  RndMeth=Zero
  R Ankle Joint Limits : Subsystem
  R BFSH : Subsystem
  R BFSH Link : Subsystem
  R GAS : Subsystem
  R GAS Link : Subsystem
  R GLU : Subsystem
  R GLU Link : Subsystem
  R HAB : Subsystem
  R HAB Link : Subsystem
  R HAD : Subsystem
  R HAD Link : Subsystem
  R HAM : Subsystem
  R HAM Muscle Spindles{1,3,6,14} (4 alike) : Gain  Gain=1/loptHAM
  R HAM Muscle Spindles{5,7,10..11} (4 alike) : Gain  Gain=1/loptSOL
  R HAM Muscle Spindles{2,4,12..13} (4 alike) : Gain  Gain=1/loptBFSH
  R HAM Muscle Spindles{8..9,15..16} (4 alike) : Gain  Gain=1/loptGAS
  R HAM Link : Subsystem
  R HFL : Subsystem
  R HFL Link : Subsystem
  R Hip Roll Joint Limits : Subsystem
  R Knee Joint Limits : Subsystem
  R L Hip Joint Limits : Subsystem
  R RF : Subsystem
  R RF Link : Subsystem
  R RF1 : Subsystem
  R SOL : Subsystem
  R SOL Link : Subsystem
  R TA : Subsystem
  R TA Link : Subsystem
  R VAS : Subsystem
  R VAS Link : Subsystem
  Sum{,1,6..7,12,16,18,22,24,26} (10 alike) : Sum  Inputs=|++
  Sum{9..10,14,23,25,27} (6 alike) : Sum  Inputs=+-
  Sum{2..4,8,11,15,19..20} (8 alike) : Sum
  Sum13 : Sum  Inputs=++|
  Sum17 : Sum  Inputs=++|
  Sum21 : Sum  Inputs=-+
  Sum5 : Sum  Inputs=-+
  tag scope: LActBFSH=global, LActGAS=global, LActGLU=global, LActHAB=global, LActHAD=global, LActHAM=global, LActHFL=global, LActRF=global, LActSOL=global, LActTA=global, LActVAS=global, LAnkleStop=global, LFactBFSH=global, LFactGAS=global, LFactGLU=global, LFactHAB=global, LFactHAD=global, LFactHAM=global, LFactHFL=global, LFactRF=global, LFactSOL=global, LFactTA=global, LFactVAS=global, LFmBFSH=global, LFmGAS=global, LFmGLU=global, LFmHAB=global, LFmHAD=global, LFmHAM=global, LFmHFL=global, LFmRF=global, LFmSOL=global, LFmTA=global, LFmVAS=global, LHipRStop=global, LHipStop=global, LKneeStop=global, LLceBFSH=global, LLceGAS=global, LLceGLU=global, LLceHAB=global, LLceHAD=global, LLceHAM=global, LLceHFL=global, LLceRF=global, LLceSOL=global, LLceTA=global, LLceVAS=global, LM12=global, LM23=global, LM34=global, LM34R=global, LVceBFSH=global, LVceGAS=global, LVceGLU=global, LVceHAB=global, LVceHAD=global, LVceHAM=global, LVceHFL=global, LVceRF=global, LVceSOL=global, LVceTA=global, LVceVAS=global, Lphi12=global, Lphi23=global, Lphi34=global, LrGASk=global, LrGLU=global, LrHAMh=global, LrHAMk=global, LrHFL=global, LrRFh=global, LrRFk=global, LrVAS=global, RActBFSH=global, RActGAS=global, RActGLU=global, RActHAB=global, RActHAD=global, RActHAM=global, RActHFL=global, RActRF=global, RActSOL=global, RActTA=global, RActVAS=global, RAnkleStop=global, RFactBFSH=global, RFactGAS=global, RFactGLU=global, RFactHAB=global, RFactHAD=global, RFactHAM=global, RFactHFL=global, RFactRF=global, RFactSOL=global, RFactTA=global, RFactVAS=global, RFmBFSH=global, RFmGAS=global, RFmGLU=global, RFmHAB=global, RFmHAD=global, RFmHAM=global, RFmHFL=global, RFmRF=global, RFmSOL=global, RFmTA=global, RFmVAS=global, RHipStop=global, RHipStopR=global, RKneeStop=global, RLceBFSH=global, RLceGAS=global, RLceGLU=global, RLceHAB=global, RLceHAD=global, RLceHAM=global, RLceHFL=global, RLceRF=global, RLceSOL=global, RLceTA=global, RLceVAS=global, RM12=global, RM23=global, RM34=global, RM34R=global, RVceBFSH=global, RVceGAS=global, RVceGLU=global, RVceHAB=global, RVceHAD=global, RVceHAM=global, RVceHFL=global, RVceRF=global, RVceSOL=global, RVceTA=global, RVceVAS=global, Rphi12=global, Rphi23=global, Rphi34=global, RrGASk=global, RrGLU=global, RrHAMh=global, RrHAMk=global, RrHFL=global, RrRFh=global, RrRFk=global, RrVAS=global
  wires:
  Demux1/1 -> L Knee Joint Limits/1(phi [rad]), L VAS Link/1(phi23 [rad]), L RF Link/2(phi23 [rad]), L HAM Link/2(phi23 [rad]), L BFSH Link/1(phi23 [rad]), L GAS Link/1(phi23 [rad]), [Lphi23]
  L SOL/1(Fmtc) -> [LFmSOL], Product/2
  L TA/2(Lce) -> L TA Muscle Spindles/1
  L TA/4(A) -> [LActTA]
  F GAS/1(Fmtc) -> [LFmGAS], Product2/1, Product3/1
  Demux/1 -> L SOL Link/1(phi12 [rad]), L TA Link/1(phi12 [rad]), L GAS Link/2(phi12 [rad]), L Ankle Joint Limits/1(phi [rad]), [Lphi12]
  [LStimTA] -> L TA/1(STIM)
  [LStimSOL] -> L SOL/1(STIM)
  [LStimHAM] -> L HAM/1(STIM)
  L HAM/1(Fmtc) -> [LFmHAM], Product9/1, Product8/1
  L HAM/2(Lce) -> R HAM Muscle Spindles1/1
  L HFL/1(Fmtc) -> [LFmHFL], Product7/2
  L HFL/2(Lce) -> L HFL Muscle Spindles/1
  [LStimHFL] -> L HFL/1(STIM)
  L GLU/1(Fmtc) -> [LFmGLU], Product6/1
  [LStimGLU] -> L GLU/1(STIM)
  Sum16/1 -> [LM34]
  Demux/2 -> L Ankle Joint Limits/2(dphi [rad/s])
  Sum9/1 -> Sum/2
  Demux1/2 -> L Knee Joint Limits/2(dphi [rad/s])
  L SOL Link/1(lmtc [m]) -> L SOL/2(lmtc [m])
  L TA Link/1(lmtc [m]) -> L TA/2(lmtc [m])
  L GAS Link/3(lever12 [m]) -> Product2/2
  L GAS Link/2(lever23 [m]) -> Product3/2, [LrGASk]
  [LStimGAS] -> F GAS/1(STIM)
  L GAS Link/1(lmtu [m]) -> F GAS/2(lmtc [m])
  L VAS Link/1(lmtu [m]) -> L VAS/2(lmtc [m])
  L HAM Link/1(lmtu [m]) -> L HAM/2(lmtc [m])
  L HAM Link/2(lever34 [m]) -> Product8/2, [LrHAMh]
  L HAM Link/3(lever23 [m]) -> Product9/2, [LrHAMk]
  Product3/1 -> Sum2/2
  Sum3/1 -> Sum14/1
  Sum4/1 -> Sum9/1
  [Lphi12dphi12] -> Demux/1
  [Lphi23dphi23] -> Demux1/1
  [Lphi34dphi34] -> Demux2/1
  Demux2/1 -> L Hip Joint Limits/1(phi [rad]), L HFL Link/1(phi34 [rad]), L GLU Link/1(phi34 [rad]), L RF Link/1(phi34 [rad]), L HAM Link/1(phi34 [rad]), [Lphi34]
  L SOL Link/2(lever [m]) -> Product/1
  Product/1 -> Sum4/2
  Product2/1 -> Sum4/1
  L TA Link/2(lever [m]) -> Product1/2
  Product1/1 -> Sum9/2
  L Ankle Joint Limits/1(M_stop [Nm]) -> Sum/1, [LAnkleStop]
  Sum/1 -> [LM12]
  L SOL/4(A) -> [LActSOL]
  F GAS/4(A) -> [LActGAS]
  L VAS/4(A) -> [LActVAS]
  L VAS/1(Fmtc) -> [LFmVAS], Product4/2
  Sum1/1 -> [LM23]
  L Knee Joint Limits/1(M_stop [Nm]) -> Sum1/1, [LKneeStop]
  Sum5/1 -> Sum1/2
  L VAS Link/2(lever [m]) -> [LrVAS], Product4/1
  Sum2/1 -> Sum5/1
  L HAM/4(A) -> [LActHAM]
  Product8/1 -> Sum3/2
  Product6/1 -> Sum3/1
  L GLU Link/1(lmtu [m]) -> L GLU/2(lmtc [m])
  L GLU Link/2(lever [m]) -> Product6/2, [LrGLU]
  L GLU/4(A) -> [LActGLU]
  Demux2/2 -> L Hip Joint Limits/2(dphi [rad/s])
  L Hip Joint Limits/1(M_stop [Nm]) -> Sum16/1, [LHipStop]
  Sum14/1 -> Sum16/2
  L HFL Link/1(lmtu [m]) -> L HFL/2(lmtc [m])
  L HFL/4(A) -> [LActHFL]
  L HFL Link/2(lever [m]) -> Product7/1, [LrHFL]
  [LStimVAS] -> L VAS/1(STIM)
  L GLU/2(Lce) -> L HFL Muscle Spindles3/1
  L GLU/3(Vce) -> L HFL Muscle Spindles2/1
  L HAM/3(Vce) -> R HAM Muscle Spindles6/1
  F GAS/3(Vce) -> R HAM Muscle Spindles9/1
  F GAS/2(Lce) -> R HAM Muscle Spindles8/1
  L SOL/2(Lce) -> R HAM Muscle Spindles10/1
  L SOL/3(Vce) -> R HAM Muscle Spindles11/1
  L TA/3(Vce) -> L TA Muscle Spindles1/1
  L VAS/3(Vce) -> L RF Muscle Spindles6/1
  L VAS/2(Lce) -> L RF Muscle Spindles4/1
  L HFL/3(Vce) -> L HFL Muscle Spindles1/1
  R RF1/4(A) -> [LActRF]
  R RF1/3(Vce) -> L RF Muscle Spindles2/1
  R RF1/2(Lce) -> L RF Muscle Spindles/1
  L RF Link/1(lmtu [m]) -> R RF1/2(lmtc [m])
  L RF Link/2(lever34 [m]) -> Product5/1, [LrRFh]
  L RF Link/3(lever23 [m]) -> Product15/1, [LrRFk]
  [LStimRF] -> R RF1/1(STIM)
  Product7/1 -> Sum11/1
  Product5/1 -> Sum11/2
  Product15/1 -> Sum17/2
  Sum17/1 -> Sum5/2
  Product4/1 -> Sum17/1
  [LStimBFSH] -> L BFSH/1(STIM)
  L BFSH Link/1(lmtu [m]) -> L BFSH/2(lmtc [m])
  L BFSH Link/2(lever [m]) -> Product20/2
  L BFSH/4(A) -> [LActBFSH]
  L BFSH/2(Lce) -> R HAM Muscle Spindles4/1
  L BFSH/3(Vce) -> R HAM Muscle Spindles2/1
  Product20/1 -> Sum22/2
  Sum22/1 -> Sum2/1
  Product9/1 -> Sum22/1
  L HFL Muscle Spindles1/1 -> [LVceHFL]
  L HFL Muscle Spindles2/1 -> [LVceGLU]
  L HFL Muscle Spindles3/1 -> [LLceGLU]
  L RF Muscle Spindles6/1 -> [LVceVAS]
  R RF1/1(Fmtc) -> [LFmRF], Product5/2, Product15/2
  L BFSH/1(Fmtc) -> Product20/1, [LFmBFSH]
  R HAM Muscle Spindles8/1 -> [LLceGAS]
  R HAM Muscle Spindles9/1 -> [LVceGAS]
  R HAM Muscle Spindles10/1 -> [LLceSOL]
  R HAM Muscle Spindles11/1 -> [LVceSOL]
  L TA/1(Fmtc) -> [LFmTA], Product1/1
  L TA Muscle Spindles1/1 -> [LVceTA]
  L HFL Muscle Spindles/1 -> [LLceHFL]
  R HAM Muscle Spindles1/1 -> [LLceHAM]
  R HAM Muscle Spindles6/1 -> [LVceHAM]
  L RF Muscle Spindles/1 -> [LLceRF]
  L RF Muscle Spindles2/1 -> [LVceRF]
  R HAM Muscle Spindles4/1 -> [LLceBFSH]
  R HAM Muscle Spindles2/1 -> [LVceBFSH]
  L RF Muscle Spindles4/1 -> [LLceVAS]
  L TA Muscle Spindles/1 -> [LLceTA]
  Demux4/1 -> R Knee Joint Limits/1(phi [rad]), R VAS Link/1(phi23 [rad]), R RF Link/2(phi23 [rad]), R HAM Link/2(phi23 [rad]), R BFSH Link/1(phi23 [rad]), R GAS Link/1(phi23 [rad]), [Rphi23]
  R SOL/1(Fmtc) -> Product10/2, [RFmSOL]
  R TA/2(Lce) -> L TA Muscle Spindles2/1
  R TA/4(A) -> [RActTA]
  R GAS/1(Fmtc) -> Product13/1, Product16/1, [RFmGAS]
  Demux3/1 -> R SOL Link/1(phi12 [rad]), R TA Link/1(phi12 [rad]), R GAS Link/2(phi12 [rad]), R Ankle Joint Limits/1(phi [rad]), [Rphi12]
  [RStimTA] -> R TA/1(STIM)
  [RStimSOL] -> R SOL/1(STIM)
  [RStimHAM] -> R HAM/1(STIM)
  R HAM/1(Fmtc) -> Product23/1, Product22/1, [RFmHAM]
  R HAM/2(Lce) -> R HAM Muscle Spindles3/1
  R HFL/1(Fmtc) -> Product21/2, [RFmHFL]
  R HFL/2(Lce) -> L HFL Muscle Spindles4/1
  [RStimHFL] -> R HFL/1(STIM)
  R GLU/1(Fmtc) -> Product19/1, [RFmGLU]
  [RStimGLU] -> R GLU/1(STIM)
  Sum12/1 -> [RM34]
  Demux3/2 -> R Ankle Joint Limits/2(dphi [rad/s])
  Sum23/1 -> Sum6/2
  Demux4/2 -> R Knee Joint Limits/2(dphi [rad/s])
  R SOL Link/1(lmtc [m]) -> R SOL/2(lmtc [m])
  R TA Link/1(lmtc [m]) -> R TA/2(lmtc [m])
  R GAS Link/3(lever12 [m]) -> Product13/2
  R GAS Link/2(lever23 [m]) -> Product16/2, [RrGASk]
  [RStimGAS] -> R GAS/1(STIM)
  R GAS Link/1(lmtu [m]) -> R GAS/2(lmtc [m])
  R VAS Link/1(lmtu [m]) -> R VAS/2(lmtc [m])
  R HAM Link/1(lmtu [m]) -> R HAM/2(lmtc [m])
  R HAM Link/2(lever34 [m]) -> Product22/2, [RrHAMh]
  R HAM Link/3(lever23 [m]) -> Product23/2, [RrHAMk]
  Product16/1 -> Sum15/2
  Sum19/1 -> Sum10/1
  Sum20/1 -> Sum23/1
  [Rphi12dphi12] -> Demux3/1
  [Rphi23dphi23] -> Demux4/1
  [Rphi34dphi34] -> Demux5/1
  Demux5/1 -> R L Hip Joint Limits/1(phi [rad]), R HFL Link/1(phi34 [rad]), R GLU Link/1(phi34 [rad]), R RF Link/1(phi34 [rad]), R HAM Link/1(phi34 [rad]), [Rphi34]
  R SOL Link/2(lever [m]) -> Product10/1
  Product10/1 -> Sum20/2
  Product13/1 -> Sum20/1
  R TA Link/2(lever [m]) -> Product11/2
  Product11/1 -> Sum23/2
  R Ankle Joint Limits/1(M_stop [Nm]) -> Sum6/1, [RAnkleStop]
  Sum6/1 -> [RM12]
  R SOL/4(A) -> [RActSOL]
  R GAS/4(A) -> [RActGAS]
  R VAS/4(A) -> [RActVAS]
  R VAS/1(Fmtc) -> Product17/2, [RFmVAS]
  Sum7/1 -> [RM23]
  R Knee Joint Limits/1(M_stop [Nm]) -> Sum7/1, [RKneeStop]
  Sum21/1 -> Sum7/2
  R VAS Link/2(lever [m]) -> [RrVAS], Product17/1
  Sum15/1 -> Sum21/1
  R HAM/4(A) -> [RActHAM]
  Product22/1 -> Sum19/2
  Product19/1 -> Sum19/1
  R GLU Link/1(lmtu [m]) -> R GLU/2(lmtc [m])
  R GLU Link/2(lever [m]) -> Product19/2, [RrGLU]
  R GLU/4(A) -> [RActGLU]
  Demux5/2 -> R L Hip Joint Limits/2(dphi [rad/s])
  R L Hip Joint Limits/1(M_stop [Nm]) -> Sum12/1, [RHipStop]
  Sum10/1 -> Sum12/2
  R HFL Link/1(lmtu [m]) -> R HFL/2(lmtc [m])
  R HFL/4(A) -> [RActHFL]
  R HFL Link/2(lever [m]) -> Product21/1, [RrHFL]
  [RStimVAS] -> R VAS/1(STIM)
  R GLU/2(Lce) -> L HFL Muscle Spindles7/1
  R GLU/3(Vce) -> L HFL Muscle Spindles6/1
  R HAM/3(Vce) -> R HAM Muscle Spindles14/1
  R GAS/3(Vce) -> R HAM Muscle Spindles16/1
  R GAS/2(Lce) -> R HAM Muscle Spindles15/1
  R SOL/2(Lce) -> R HAM Muscle Spindles5/1
  R SOL/3(Vce) -> R HAM Muscle Spindles7/1
  R TA/3(Vce) -> L TA Muscle Spindles3/1
  R VAS/3(Vce) -> L RF Muscle Spindles7/1
  R VAS/2(Lce) -> L RF Muscle Spindles5/1
  R HFL/3(Vce) -> L HFL Muscle Spindles5/1
  R RF/4(A) -> [RActRF]
  R RF/3(Vce) -> L RF Muscle Spindles3/1
  R RF/2(Lce) -> L RF Muscle Spindles1/1
  R RF Link/1(lmtu [m]) -> R RF/2(lmtc [m])
  R RF Link/2(lever34 [m]) -> Product18/1, [RrRFh]
  R RF Link/3(lever23 [m]) -> Product12/1, [RrRFk]
  [RStimRF] -> R RF/1(STIM)
  Sum8/1 -> Sum10/2
  Product21/1 -> Sum8/1
  Product18/1 -> Sum8/2
  Product12/1 -> Sum13/2
  Sum13/1 -> Sum21/2
  Product17/1 -> Sum13/1
  [RStimBFSH] -> R BFSH/1(STIM)
  R BFSH Link/1(lmtu [m]) -> R BFSH/2(lmtc [m])
  R BFSH Link/2(lever [m]) -> Product14/2
  R BFSH/4(A) -> [RActBFSH]
  R BFSH/2(Lce) -> R HAM Muscle Spindles13/1
  R BFSH/3(Vce) -> R HAM Muscle Spindles12/1
  Product14/1 -> Sum18/2
  Sum18/1 -> Sum15/1
  Product23/1 -> Sum18/1
  L HFL Muscle Spindles5/1 -> [RVceHFL]
  L HFL Muscle Spindles6/1 -> [RVceGLU]
  L HFL Muscle Spindles7/1 -> [RLceGLU]
  L RF Muscle Spindles7/1 -> [RVceVAS]
  R RF/1(Fmtc) -> Product18/2, Product12/2, [RFmRF]
  R BFSH/1(Fmtc) -> Product14/1, [RFmBFSH]
  R HAM Muscle Spindles15/1 -> [RLceGAS]
  R HAM Muscle Spindles16/1 -> [RVceGAS]
  R HAM Muscle Spindles5/1 -> [RLceSOL]
  R HAM Muscle Spindles7/1 -> [RVceSOL]
  R TA/1(Fmtc) -> Product11/1, [RFmTA]
  L TA Muscle Spindles3/1 -> [RVceTA]
  L HFL Muscle Spindles4/1 -> [RLceHFL]
  R HAM Muscle Spindles3/1 -> [RLceHAM]
  R HAM Muscle Spindles14/1 -> [RVceHAM]
  L RF Muscle Spindles1/1 -> [RLceRF]
  L RF Muscle Spindles3/1 -> [RVceRF]
  R HAM Muscle Spindles13/1 -> [RLceBFSH]
  R HAM Muscle Spindles12/1 -> [RVceBFSH]
  L RF Muscle Spindles5/1 -> [RLceVAS]
  L TA Muscle Spindles2/1 -> [RLceTA]
  Sum11/1 -> Sum14/2
  [LStimHAD] -> L HAD/1(STIM)
  [LStimHAB] -> L HAB/1(STIM)
  Sum26/1 -> [LM34R]
  [Lphi34dphi34R] -> Demux6/1
  Demux6/1 -> L HAB Link/1(phi34R [rad]), L HAD Link/1(phi34R [rad]), L Hip Roll Joint Limits/1(phi [rad])
  Product26/1 -> Sum25/1
  L HAB Link/1(lmtu [m]) -> L HAB/2(lmtc [m])
  L HAB Link/2(lever [m]) -> Product26/2
  Demux6/2 -> L Hip Roll Joint Limits/2(dphi [rad/s])
  L Hip Roll Joint Limits/1(M_stop [Nm]) -> Sum26/1, [LHipRStop]
  Sum25/1 -> Sum26/2
  Product27/1 -> Sum25/2
  L HAD Link/1(lmtu [m]) -> L HAD/2(lmtc [m])
  L HAD Link/2(lever [m]) -> Product27/1
  [RStimHAD] -> R HAD/1(STIM)
  Sum24/1 -> [RM34R]
  [Rphi34dphi34R] -> Demux7/1
  Demux7/1 -> R HAD Link/1(phi34R [rad]), R HAB Link/1(phi34R [rad]), R Hip Roll Joint Limits/1(phi [rad])
  Product24/1 -> Sum27/1
  R HAB Link/1(lmtu [m]) -> R HAB/2(lmtc [m])
  R HAB Link/2(lever [m]) -> Product24/2
  Demux7/2 -> R Hip Roll Joint Limits/2(dphi [rad/s])
  R Hip Roll Joint Limits/1(M_stop [Nm]) -> Sum24/1, [RHipStopR]
  Sum27/1 -> Sum24/2
  Product25/1 -> Sum27/2
  R HAD Link/1(lmtu [m]) -> R HAD/2(lmtc [m])
  R HAD Link/2(lever [m]) -> Product25/1
  [RStimHAB] -> R HAB/1(STIM)
  L HAB/4(A) -> [LActHAB]
  L HAB/2(Lce) -> L HFL Muscle Spindles10/1
  L HAB/3(Vce) -> L HFL Muscle Spindles9/1
  L HFL Muscle Spindles9/1 -> [LVceHAB]
  L HFL Muscle Spindles10/1 -> [LLceHAB]
  L HAB/1(Fmtc) -> Product26/1, [LFmHAB]
  L HFL Muscle Spindles8/1 -> [LVceHAD]
  L HFL Muscle Spindles11/1 -> [LLceHAD]
  L HAD/2(Lce) -> L HFL Muscle Spindles11/1
  L HAD/3(Vce) -> L HFL Muscle Spindles8/1
  L HAD/4(A) -> [LActHAD]
  L HAD/1(Fmtc) -> Product27/2, [LFmHAD]
  R HAB/4(A) -> [RActHAB]
  R HAB/2(Lce) -> L HFL Muscle Spindles13/1
  R HAB/3(Vce) -> L HFL Muscle Spindles12/1
  L HFL Muscle Spindles12/1 -> [RVceHAB]
  L HFL Muscle Spindles13/1 -> [RLceHAB]
  R HAB/1(Fmtc) -> [RFmHAB], Product24/1
  L HFL Muscle Spindles14/1 -> [RVceHAD]
  L HFL Muscle Spindles15/1 -> [RLceHAD]
  R HAD/2(Lce) -> L HFL Muscle Spindles15/1
  R HAD/3(Vce) -> L HFL Muscle Spindles14/1
  R HAD/4(A) -> [RActHAD]
  R HAD/1(Fmtc) -> [RFmHAD], Product25/2
  R HFL/5(Fac) -> [RFactHFL]
  R HAD/5(Fac) -> [RFactHAD]
  R HAB/5(Fac) -> [RFactHAB]
  R RF/5(Fac) -> [RFactRF]
  R VAS/5(Fac) -> [RFactVAS]
  R TA/5(Fac) -> [RFactTA]
  R SOL/5(Fac) -> [RFactSOL]
  R GAS/5(Fac) -> [RFactGAS]
  R BFSH/5(Fac) -> [RFactBFSH]
  R HAM/5(Fac) -> [RFactHAM]
  R GLU/5(Fac) -> [RFactGLU]
  L TA/5(Fac) -> [LFactTA]
  L SOL/5(Fac) -> [LFactSOL]
  F GAS/5(Fac) -> [LFactGAS]
  L VAS/5(Fac) -> [LFactVAS]
  L BFSH/5(Fac) -> [LFactBFSH]
  L HAM/5(Fac) -> [LFactHAM]
  R RF1/5(Fac) -> [LFactRF]
  L HFL/5(Fac) -> [LFactHFL]
  L GLU/5(Fac) -> [LFactGLU]
  L HAB/5(Fac) -> [LFactHAB]
  L HAD/5(Fac) -> [LFactHAD]
